simulink model "Lagaya_RJ_MATLAB_No1_Reduced"  (R2024a)
settings: Solver=VariableStepAuto  StartTime=0.0  StopTime=10.0  RelTol=1e-3
settings Model: Creator=Vincent L. Alcantara  LastModifiedBy=Rod Joshua Lagaya
settings RTWCC: GPUComputeCapability=3.5

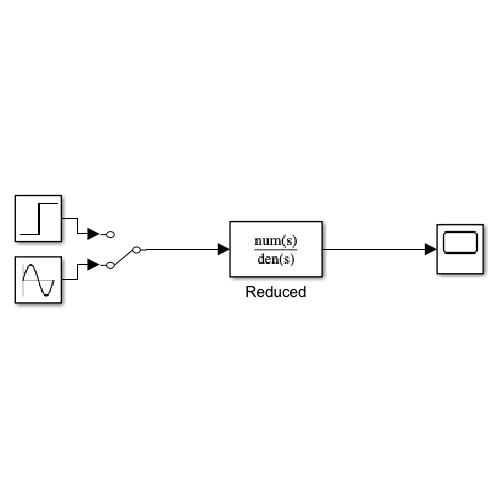
[thumbnail: Simulink's stored preview of the top-level diagram]
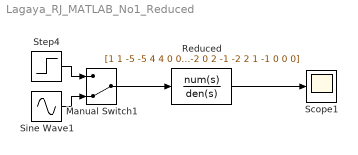
== system Lagaya_RJ_MATLAB_No1_Reduced ==
  Manual Switch1 : ManualSwitch  CurrentSetting=0
  Reduced : TransferFcn  Numerator=[1 1 -5 -5 4 4 0 0 0 0]  Denominator=[1 0 -2 0 2 -1 -2 2 1 -1 0 0 0]
  Scope1 : Scope
  Sine Wave1 : Sin  SampleTime=0
  Step4 : Step  Time=0  SampleTime=0
  wires:
  Sine Wave1/1 -> Manual Switch1/2
  Step4/1 -> Manual Switch1/1
  Manual Switch1/1 -> Reduced/1
  Reduced/1 -> Scope1/1
